simulink model "one_gen_model"  (R2022a)
settings: Solver=VariableStepAuto  StartTime=0.0  StopTime=t_final  MaxStep=t_max_step  RelTol=1e-3
values from neighbouring files (symbols this model uses):
  a_21 = (12e3)^2 * abs(-1 / (1j * ws * 0.0275))    [main.m]    (also in main_one_gen.m = (12e3)^2 * abs(1 / (1j * ws * 0.0275)); main_two_gen.m = (12e3)^2 * abs(1 / (1j * ws * 0.0275)); one_gen_model_sim.m = (12e3)^2 * abs(-1/(1j*ws*0.0275)))
  D = 0.18 * K    (= 1.5714e-07)    [main.m]    (also in main_one_gen.m = 1.5714e-08; one_gen_model_sim.m)
  d_0 = d2_array(ii)    [main_one_gen.m]    (also in one_gen_model_sim.m = -1.25663706144)
  K = 8.73e-7    (= 8.73e-07)    [main.m]    (also in main_one_gen.m = 8.73e-08; one_gen_model_sim.m = k_array(ii))
  P_L = -5e6    (= -5000000)    [one_gen_model_sim.m]
  P_ref = 4e6    (= 4000000)    [main.m]    (also in main_one_gen.m = 10000000; one_gen_model_sim.m)
  w_0 = w_array(ij)    [main_one_gen.m]    (also in one_gen_model_sim.m = 307.876080052)
  ws = 50 * 2 * pi    (= 314.159265359)    [main.m]    (also in main_one_gen.m; main_two_gen.m; one_gen_model_sim.m)
settings Model: Creator=Liraz  LastModifiedBy=Liraz

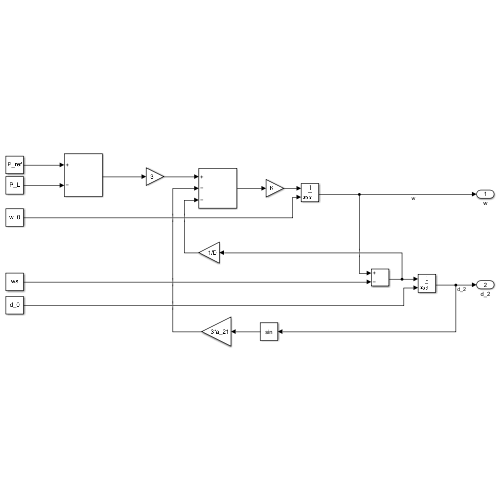
[thumbnail: Simulink's stored preview of the top-level diagram]
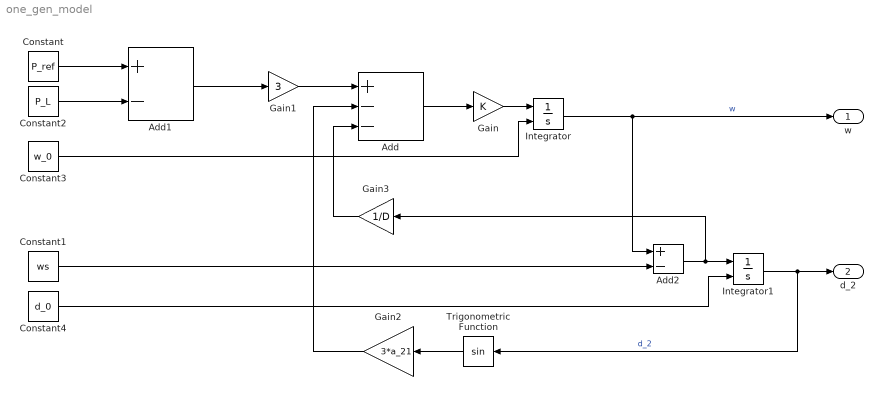
== system one_gen_model ==
  Add : Sum  Inputs=+--
  Add1 : Sum  Inputs=+-
  Add2 : Sum  Inputs=+-
  Constant : Constant  Value=P_ref
  Constant1 : Constant  Value=ws
  Constant2 : Constant  Value=P_L
  Constant3 : Constant  Value=w_0
  Constant4 : Constant  Value=d_0
  Gain : Gain  Gain=K
  Gain1 : Gain  Gain=3
  Gain2 : Gain  Gain=3*a_21
  Gain3 : Gain  Gain=1/D
  Integrator : Integrator  InitialConditionSource=external
  Integrator1 : Integrator  InitialConditionSource=external
  Trigonometric Function : Trigonometry
  w : Outport
  d_2 : Outport  Port=2
  wires:
  Gain/1 -> Integrator/1
  Constant/1 -> Add1/1
  Constant2/1 -> Add1/2
  Add1/1 -> Gain1/1
  Gain1/1 -> Add/1
  Integrator/1 -> w/1, Add2/1  "w"
  Add/1 -> Gain/1
  Trigonometric Function/1 -> Gain2/1
  Integrator1/1 -> d_2/1, Trigonometric Function/1  "d_2"
  Add2/1 -> Gain3/1, Integrator1/1
  Constant1/1 -> Add2/2
  Gain2/1 -> Add/2
  Gain3/1 -> Add/3
  Constant4/1 -> Integrator1/2
  Constant3/1 -> Integrator/2
